simulink model "Open_loop_Closed_loop_CS"  (R2023b)
settings: Solver=VariableStepAuto  StartTime=0.0  StopTime=50  RelTol=1e-3
libraries: simulink x2
settings Model: Creator=Simranprakashjagtap  LastModifiedBy=Simranprakashjagtap
settings ModelReferenceCC: EnableRefExpFcnMdlSchedulingChecks=on

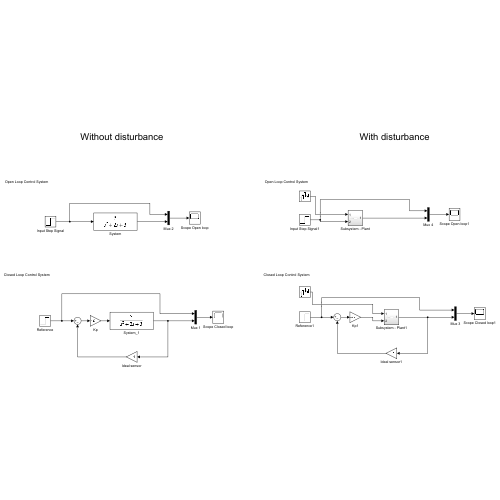
[thumbnail: Simulink's stored preview of the top-level diagram]
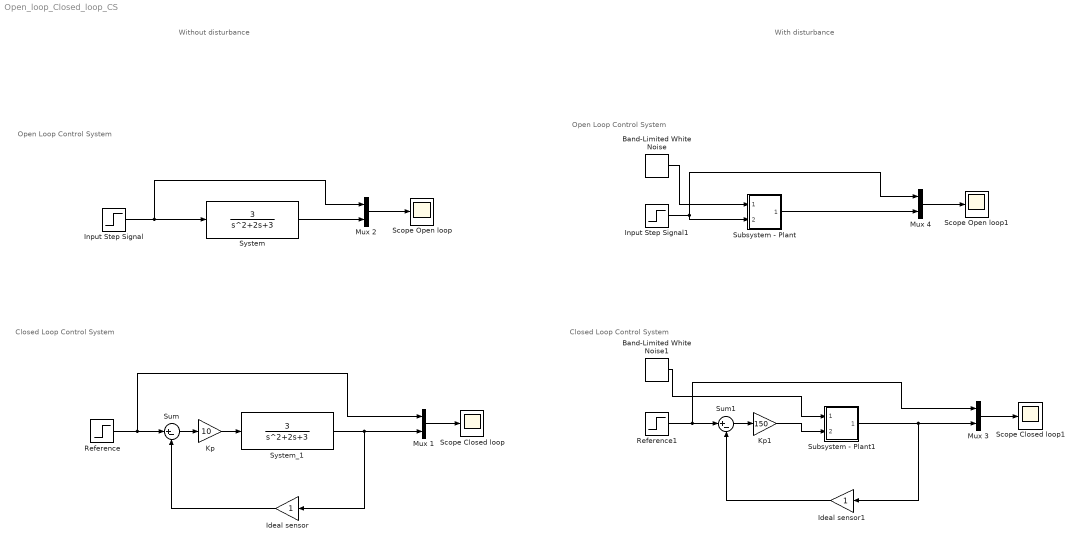
== system Open_loop_Closed_loop_CS ==
  note: With disturbance
  note: Closed Loop Control System
  note: Open Loop Control System
  note: Open Loop Control System
  note: Closed Loop Control System
  note: Without disturbance
  Band-Limited White Noise : simulink/Sources/Band-Limited White Noise  Cov=[0.1]  Ts=0.1  seed=[23341]
  Band-Limited White Noise1 : simulink/Sources/Band-Limited White Noise  Cov=[0.1]  Ts=0.1  seed=[23341]
  Ideal sensor : Gain
  Ideal sensor1 : Gain
  Input Step Signal : Step  SampleTime=0
  Input Step Signal1 : Step  SampleTime=0
  Kp : Gain  Gain=10
  Kp1 : Gain  Gain=150
  Mux {1..4} (4 alike) : Mux  Inputs=2
  Reference : Step  SampleTime=0
  Reference1 : Step  SampleTime=0
  Scope Closed loop : Scope
  Scope Closed loop1 : Scope
  Scope Open loop : Scope
  Scope Open loop1 : Scope
  Subsystem - Plant : Subsystem
  Subsystem - Plant1 : Subsystem
  Sum : Sum  Inputs=|+-
  Sum1 : Sum  Inputs=|+-
  System : TransferFcn  Numerator=[3]  Denominator=[1 2 3]
  System_1 : TransferFcn  Numerator=[3]  Denominator=[1 2 3]
  wires:
  Mux 2/1 -> Scope Open loop/1
  System/1 -> Mux 2/2
  Input Step Signal/1 -> Mux 2/1, System/1
  Ideal sensor/1 -> Sum/2
  System_1/1 -> Mux 1/2, Ideal sensor/1
  Sum/1 -> Kp/1
  Mux 1/1 -> Scope Closed loop/1
  Reference/1 -> Mux 1/1, Sum/1
  Kp/1 -> System_1/1
  Kp1/1 -> Subsystem - Plant1/2(In2)
  Reference1/1 -> Mux 3/1, Sum1/1
  Mux 3/1 -> Scope Closed loop1/1
  Sum1/1 -> Kp1/1
  Ideal sensor1/1 -> Sum1/2
  Mux 4/1 -> Scope Open loop1/1
  Input Step Signal1/1 -> Subsystem - Plant/2(In2), Mux 4/1
  Subsystem - Plant1/1(Out1) -> Mux 3/2, Ideal sensor1/1
  Band-Limited White Noise/1 -> Subsystem - Plant/1(In1)
  Subsystem - Plant/1(Out1) -> Mux 4/2
  Band-Limited White Noise1/1 -> Subsystem - Plant1/1(In1)

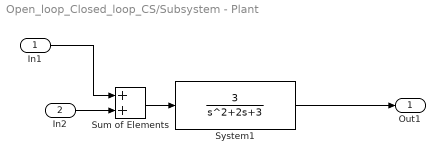
== system Open_loop_Closed_loop_CS/Subsystem - Plant ==
  In1 : Inport
  In2 : Inport  Port=2
  Sum of Elements : Sum
  System1 : TransferFcn  Numerator=[3]  Denominator=[1 2 3]
  Out1 : Outport
  wires:
  Sum of Elements/1 -> System1/1
  In2/1 -> Sum of Elements/2
  System1/1 -> Out1/1
  In1/1 -> Sum of Elements/1

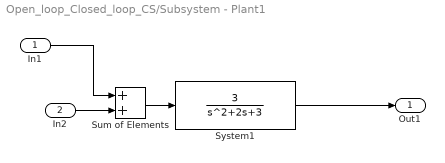
== system Open_loop_Closed_loop_CS/Subsystem - Plant1 ==
  In1 : Inport
  In2 : Inport  Port=2
  Sum of Elements : Sum
  System1 : TransferFcn  Numerator=[3]  Denominator=[1 2 3]
  Out1 : Outport
  wires:
  Sum of Elements/1 -> System1/1
  In2/1 -> Sum of Elements/2
  System1/1 -> Out1/1
  In1/1 -> Sum of Elements/1
